simulink model "LQG_sim"  (R2022b)
settings: Solver=VariableStepAuto  StartTime=0.0  StopTime=10.0  RelTol=1e-3
values from neighbouring files (symbols this model uses):
  A = [-0.051 0 -0.144 -0.056 0 0 0 0 0 0 0 0 ... (169 elements, 13x13)]    [Elicottero.mat]
  B = [0 0 0 0 0 0 0.68 3.043 0 0 0 0 ... (52 elements, 13x4)]    [Elicottero.mat]
undefined symbols (not defined in the file or in its folder): A_k, B_k, BandWidth, C, C_k, D, D_k, K_i_lq, K_s_lq, Qt, x0_obs
libraries: simulink x2
settings Model: Creator=valen  LastModifiedBy=valen

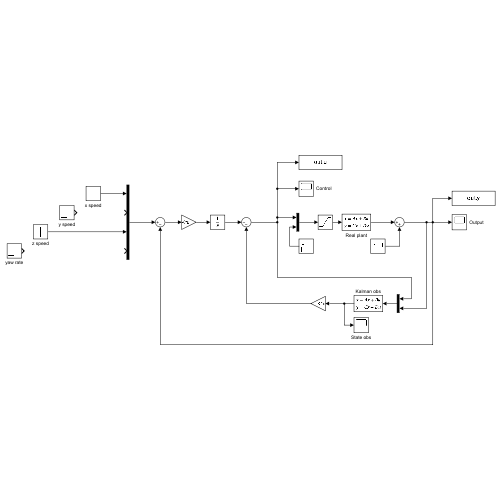
[thumbnail: Simulink's stored preview of the top-level diagram]
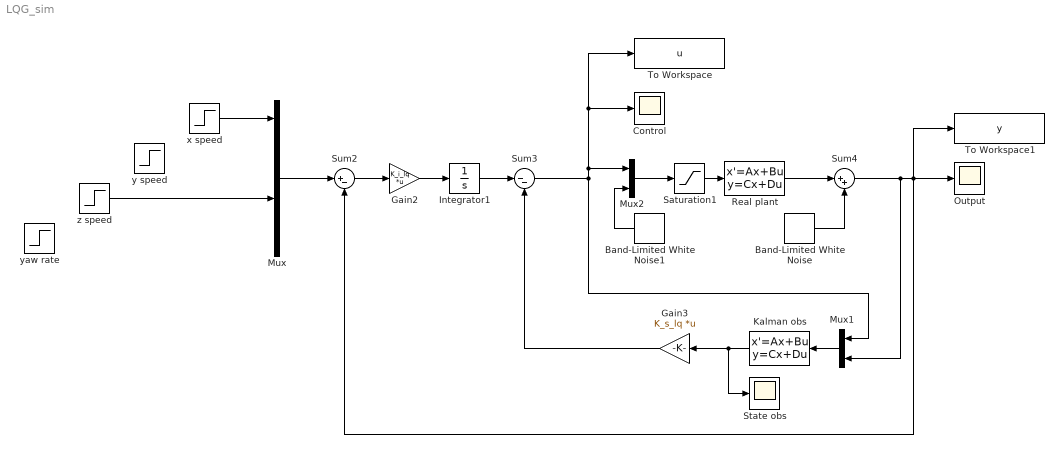
== system LQG_sim ==
  Band-Limited White Noise : simulink/Sources/Band-Limited White Noise  Cov=NoisePower  Ts=1/BandWidth  seed=[23341]
  Band-Limited White Noise1 : simulink/Sources/Band-Limited White Noise  Cov=diag(Qt)  Ts=1/BandWidth  seed=[23341]
  Control : Scope
  Gain2 : Gain  Gain=K_i_lq  Multiplication=Matrix(K*u)
  Gain3 : Gain  Gain=K_s_lq  Multiplication=Matrix(K*u)
  Integrator1 : Integrator
  Kalman obs : StateSpace  A=A_k  B=B_k  C=C_k  D=D_k  InitialCondition=0
  Mux : Mux
  Mux1 : Mux  Inputs=2
  Mux2 : Mux  Inputs=2
  Output : Scope
  Real plant : StateSpace  A=A  B=[B, eye(13)]  C=C  D=[D, zeros(4,13)]  InitialCondition=x0_obs
  Saturation1 : Saturate  UpperLimit=1  LowerLimit=-1
  State obs : Scope
  Sum2 : Sum  Inputs=|+-
  Sum3 : Sum  Inputs=|--
  Sum4 : Sum  Inputs=|++
  To Workspace : ToWorkspace  VariableName=u  SaveFormat=Structure With Time  SampleTime=-1
  To Workspace1 : ToWorkspace  VariableName=y  SaveFormat=Structure With Time  SampleTime=-1
  x speed : Step  Time=0  SampleTime=0
  y speed : Step  Time=0  SampleTime=0
  yaw rate : Step  Time=0  SampleTime=0
  z speed : Step  Time=3  After=0.5  SampleTime=0
  wires:
  z speed/1 -> Mux/3
  x speed/1 -> Mux/1
  Mux2/1 -> Saturation1/1
  Sum2/1 -> Gain2/1
  Kalman obs/1 -> State obs/1, Gain3/1
  Band-Limited White Noise/1 -> Sum4/2
  Sum4/1 -> To Workspace1/1, Output/1, Sum2/2, Mux1/2
  Real plant/1 -> Sum4/1
  Mux1/1 -> Kalman obs/1
  Integrator1/1 -> Sum3/1
  Gain3/1 -> Sum3/2
  Gain2/1 -> Integrator1/1
  Sum3/1 -> Mux2/1, To Workspace/1, Control/1, Mux1/1
  Band-Limited White Noise1/1 -> Mux2/2
  Saturation1/1 -> Real plant/1
  Mux/1 -> Sum2/1
